simulink model "model_simulation_2020a"  (R2020a)
settings: Solver=VariableStepAuto  StartTime=0.0  StopTime=0.2  RelTol=1e-3
values from neighbouring files (symbols this model uses):
  a0 = C_tustin.Numerator{1}(3)    [PID_design.m]
  a1 = C_tustin.Numerator{1}(2)    [PID_design.m]
  a2 = C_tustin.Numerator{1}(1)    [PID_design.m]
  b0 = C_tustin.Denominator{1}(3)    [PID_design.m]
  b1 = C_tustin.Denominator{1}(2)    [PID_design.m]
  b2 = C_tustin.Denominator{1}(1)    [PID_design.m]
  C_tustin = tf(C_tustin)    [PID_design.m]
  L = 0.001    [PID_design.m]
  R = 0.1    [PID_design.m]
  Ts = 0.5*10^(-3)    (= 0.0005)    [PID_design.m]
undefined symbols (not defined in the file or in its folder): dspblkCoreblockFVToolHelper, gcbh
settings Model: Creator=pmpob  LastModifiedBy=14126181
settings DebuggingCC: UnconnectedInputMsg=none  UnconnectedOutputMsg=none  UnconnectedLineMsg=none
settings ModelReferenceCC: EnableRefExpFcnMdlSchedulingChecks=off
settings RTWCC: Description=Generic Real-Time Target

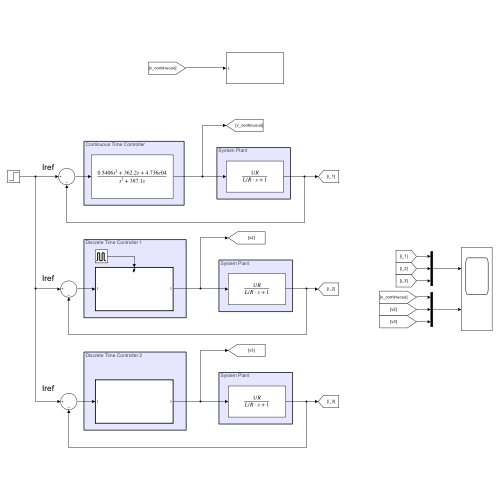
[thumbnail: Simulink's stored preview of the top-level diagram]
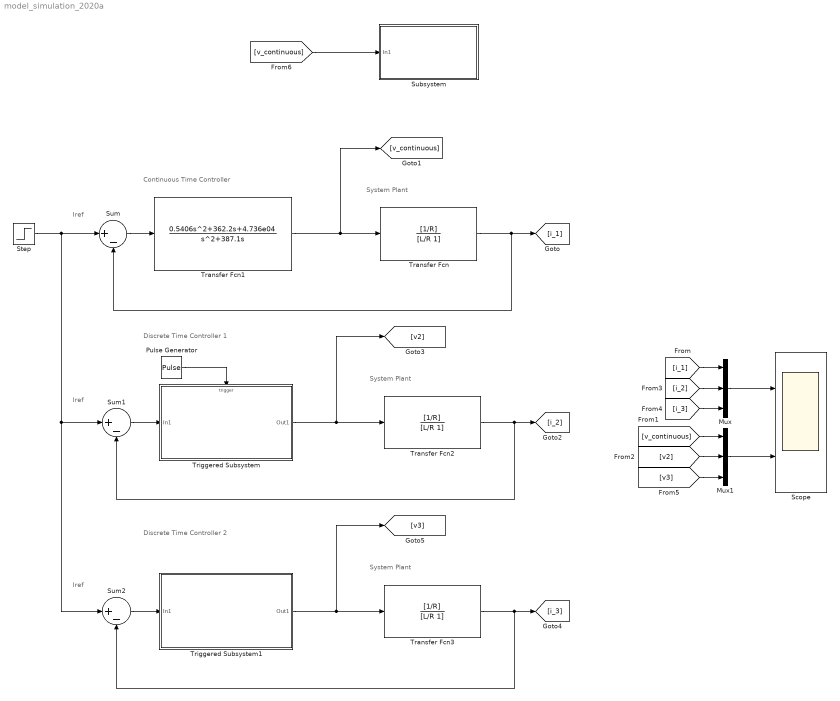
== system model_simulation_2020a ==
  note: Iref
  note: Continuous Time Controller
  note: System Plant
  note: Discrete Time Controller 1
  note: System Plant
  note: System Plant
  note: Discrete Time Controller 2
  note: Iref
  note: Iref
  Mux : Mux  Inputs=3
  Mux1 : Mux  Inputs=3
  Pulse Generator : DiscretePulseGenerator  PulseType=Time based  Period=Ts  PulseWidth=50
  Scope : Scope  NumInputPorts=2
  Step : Step  Time=0.1  SampleTime=Ts
  Subsystem : Subsystem
  Sum : Sum  Inputs=|+-
  Sum1 : Sum  Inputs=|+-
  Sum2 : Sum  Inputs=|+-
  Transfer Fcn : TransferFcn  Numerator=[1/R]  Denominator=[L/R 1]
  Transfer Fcn1 : TransferFcn  Numerator=[0.5406 362.2 4.736e04]  Denominator=[1 387.1 0]
  Transfer Fcn2 : TransferFcn  Numerator=[1/R]  Denominator=[L/R 1]
  Transfer Fcn3 : TransferFcn  Numerator=[1/R]  Denominator=[L/R 1]
  Triggered Subsystem : Subsystem  TreatAsAtomicUnit=on
  Triggered Subsystem1 : Subsystem  TreatAsAtomicUnit=on
  wires:
  Transfer Fcn1/1 -> [v_continuous], Transfer Fcn/1
  Sum/1 -> Transfer Fcn1/1
  Transfer Fcn/1 -> [i_1], Sum/2
  Mux/1 -> Scope/1
  [i_1] -> Mux/1
  Mux1/1 -> Scope/2
  [v_continuous] -> Mux1/1
  Sum1/1 -> Triggered Subsystem/1(In1)
  Transfer Fcn2/1 -> Sum1/2, [i_2]
  Triggered Subsystem/1(Out1) -> [v2], Transfer Fcn2/1
  [v2] -> Mux1/2
  [i_2] -> Mux/2
  Pulse Generator/1 -> Triggered Subsystem/Trigger
  Triggered Subsystem1/1(Out1) -> [v3], Transfer Fcn3/1
  Step/1 -> Sum2/1, Sum1/1, Sum/1
  Sum2/1 -> Triggered Subsystem1/1(In1)
  Transfer Fcn3/1 -> Sum2/2, [i_3]
  [i_3] -> Mux/3
  [v3] -> Mux1/3
  [v_continuous] -> Subsystem/1(In1)

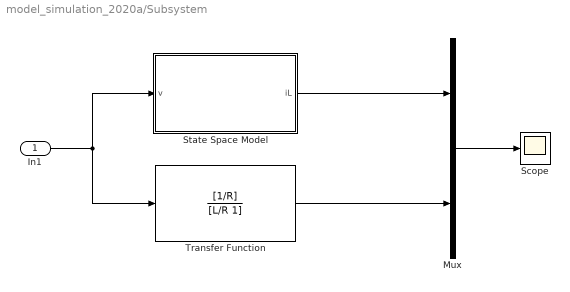
== system model_simulation_2020a/Subsystem ==
  In1 : Inport
  Mux : Mux  Inputs=2
  Scope : Scope
  State Space Model : Subsystem
  Transfer Function : TransferFcn  Numerator=[1/R]  Denominator=[L/R 1]
  wires:
  In1/1 -> Transfer Function/1, State Space Model/1(v)
  Mux/1 -> Scope/1
  Transfer Function/1 -> Mux/2
  State Space Model/1(iL) -> Mux/1

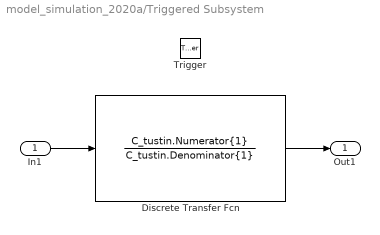
== system model_simulation_2020a/Triggered Subsystem ==
  In1 : Inport
  Trigger : TriggerPort  VariantControl=(inherit)
  Discrete Transfer Fcn : DiscreteTransferFcn  LoadFcn=dspblkCoreblockFVToolHelper(gcbh,'load');  Numerator=C_tustin.Numerator{1}  Denominator=C_tustin.Denominator{1}
      settings: CopyFcn=dspblkCoreblockFVToolHelper(gcbh,'copy');  DeleteFcn=dspblkCoreblockFVToolHelper(gcbh,'close');  ModelCloseFcn=dspblkCoreblockFVToolHelper(gcbh,'close');  PreSaveFcn=dspblkCoreblockFVToolHelper(gcbh,'presave');  PostSaveFcn=dspblkCoreblockFVToolHelper(gcbh,'postsave');  CloseFcn=dspblkCoreblockFVToolHelper(gcbh,'close');
  Out1 : Outport
  wires:
  Discrete Transfer Fcn/1 -> Out1/1
  In1/1 -> Discrete Transfer Fcn/1

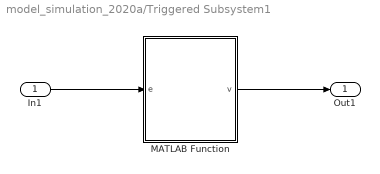
== system model_simulation_2020a/Triggered Subsystem1 ==
  In1 : Inport
  MATLAB Function : MATLAB Function  TreatAsAtomicUnit=on
  Out1 : Outport
  wires:
  MATLAB Function/1(v) -> Out1/1
  In1/1 -> MATLAB Function/1(e)

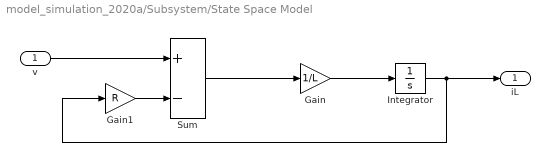
== system model_simulation_2020a/Subsystem/State Space Model ==
  v : Inport
  Gain : Gain  Gain=1/L
  Gain1 : Gain  Gain=R
  Integrator : Integrator
  Sum : Sum  Inputs=+-
  iL : Outport
  wires:
  Gain/1 -> Integrator/1
  Integrator/1 -> Gain1/1, iL/1
  v/1 -> Sum/1
  Sum/1 -> Gain/1
  Gain1/1 -> Sum/2

== matlab function model_simulation_2020a/Triggered Subsystem1/MATLAB Function ==
  settings: updateMethod=DISCRETE  sampleTime=Ts
  data: e input; v output; a0 parameter; a1 parameter; a2 parameter; b0 parameter; b1 parameter; b2 parameter
function v = fcn(e, a0, a1, a2, b0, b1, b2)

% variables that are stored in memmory
persistent e1 e2 v1 v2

% init controller
if isempty(e1)
    e1 = 0;
    e2 = 0;
    v1 = 0;
    v2 = 0;
end

% controller
v = e*(a2/b2) + e1*(a1/b2) + e2*(a0/b2) ...
  - v1*(b1/b2) - v2*(b0/b2);

% save variables
e2 = e1;
e1 = e;

v2 = v1;
v1 = v;
